simulink model "dmpwalk2014"  (R2018b)
settings: Solver=VariableStepAuto  StartTime=0.0  StopTime=100  RelTol=1e-3
values from neighbouring files (symbols this model uses):
  arm_radius = leg_radius    (= 0.01)    [Nao_paramter.m]
  foot_height = 0.02    [Nao_paramter.m]
  foot_length = 0.1    [Nao_paramter.m]
  foot_mass = 0.17184    [Nao_paramter.m]
  foot_width = 0.05    [Nao_paramter.m]
  ground_height = 0.0025    [Nao_paramter.m]
  ground_length = 5    [Nao_paramter.m]
  ground_width = 2    [Nao_paramter.m]
  hand_mass = 0.18533    [Nao_paramter.m]
  head_mass = 0.60533    [Nao_paramter.m]
  hip_mass = 0.14053    [Nao_paramter.m]
  hip_off_Y = 0.05    [Nao_paramter.m]
  hip_off_Z = 0.085    [Nao_paramter.m]
  leg_radius = 0.01    [Nao_paramter.m]
  lowerarm_length = 0.05595    [Nao_paramter.m]
  lowerarm_mass = 0.07761    [Nao_paramter.m]
  neck_length = 0.03    [Nao_paramter.m]
  neck_mass = 0.07842    [Nao_paramter.m]
  neck_off_Z = 0.1265    [Nao_paramter.m]
  shoulder_mass = 0.09304    [Nao_paramter.m]
  thigh_mass = 0.38968    [Nao_paramter.m]
  tibia_mass = 0.30142    [Nao_paramter.m]
  torso_height = foot_height + tibia_length + thigh_length + 0.5*hip_off_Z    (= 0.2654)    [Nao_paramter.m]
  torso_mass = 1.0496    [Nao_paramter.m]
  upperarm_length = 0.105    [Nao_paramter.m]
  upperarm_mass = 0.15777    [Nao_paramter.m]
undefined symbols (not defined in the file or in its folder): sigbuilder_block, X, Y, Z
libraries: sm_lib x87, nesl_utility x15, Contact_Forces_Lib x10
(part 1 of 5)
settings Model: Creator=zicho  LastModifiedBy=zicho

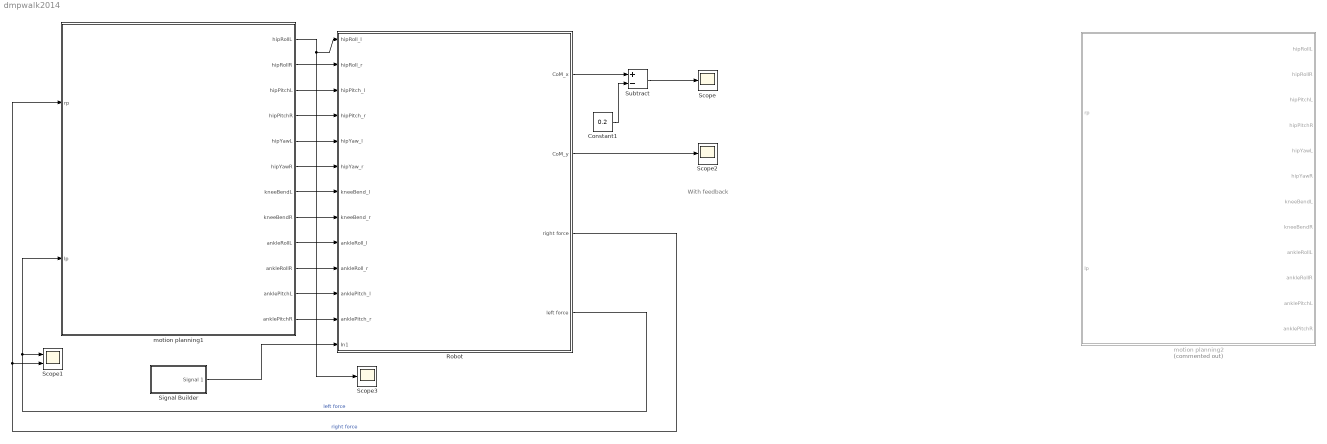
== system dmpwalk2014 ==
  note: With feedback
  Constant1 : Constant  Value=0.2
  Robot : Subsystem
      mask Display: image('multibody.jpg');
  Scope : Scope
  Scope1 : Scope  NumInputPorts=2
  Scope2 : Scope
  Scope3 : Scope
  Signal Builder : Subsystem  Tag=STV Subsys  LoadFcn=sigbuilder_block('load',[437.6 199.2 550.4 400 ]);  StartFcn=sigbuilder_block('start');  StopFcn=sigbuilder_block('stop');  ClipboardFcn=sigbuilder_block('clipboard');  mask(Sigbuilder block){tuvar=[0:10]}
      mask help: Simulink:masks:SigbuilderBlock_MD
      mask init:
      | if ~strcmp(get_param(bdroot(gcbh),'SimulationStatus'),'stopped') tuvar = sigbuilder_block('maskInit'); end
      settings: CopyFcn=sigbuilder_block('copy');  DeleteFcn=sigbuilder_block('delete');  ModelCloseFcn=sigbuilder_block('modelClose');  PreSaveFcn=sigbuilder_block('preSave');  PauseFcn=sigbuilder_block('pause');  ContinueFcn=sigbuilder_block('continue');  NameChangeFcn=sigbuilder_block('namechange');  OpenFcn=sigbuilder_block('open',[437.6 199.2 550.4 400 ]);  CloseFcn=sigbuilder_block('close');
      mask Display: plot(0, 0, 100, 100,[2, 2, 32, 32, 2], [68, 8, 8, 68, 68],[32, 2], [38, 38], [32, 19, 2],[53, 60, 44], [32, 17, 17, 2],[16, 16, 31, 31]);txt = getActiveGroup(gcbh);text(2, 100, txt,'verticalAlignment', 'top');
  Subtract : Sum  Inputs=+-
  motion planning1 : Stateflow chart  TreatAsAtomicUnit=on
  motion planning2 : Stateflow chart  Commented=on  TreatAsAtomicUnit=on
  wires:
  Signal Builder/1(Signal 1) -> Robot/13(In1)
  motion planning1/10(ankleRollR) -> Robot/10(ankleRoll_r)
  motion planning1/9(ankleRollL) -> Robot/9(ankleRoll_l)
  motion planning1/8(kneeBendR) -> Robot/8(kneeBend_r)
  Robot/4(left force) -> Scope1/1, motion planning1/2(lp)  "left force"
  Robot/3(right force) -> motion planning1/1(rp), Scope1/2  "right force"
  Subtract/1 -> Scope/1
  motion planning1/2(hipRollR) -> Robot/2(hipRoll_r)
  motion planning1/1(hipRollL) -> Scope3/1, Robot/1(hipRoll_l)
  motion planning1/7(kneeBendL) -> Robot/7(kneeBend_l)
  Robot/1(CoM_x) -> Subtract/1
  motion planning1/5(hipYawL) -> Robot/5(hipYaw_l)
  motion planning1/6(hipYawR) -> Robot/6(hipYaw_r)
  Robot/2(CoM_y) -> Scope2/1
  motion planning1/11(anklePitchL) -> Robot/11(anklePitch_l)
  motion planning1/12(anklePitchR) -> Robot/12(anklePitch_r)
  Constant1/1 -> Subtract/2
  motion planning1/4(hipPitchR) -> Robot/4(hipPitch_r)
  motion planning1/3(hipPitchL) -> Robot/3(hipPitch_l)
